simulink model "Rover_Simulation_R2023b"  (R2023b)
settings: Solver=VariableStepAuto  StartTime=0.0  StopTime=500  MaxStep=1e-1  RelTol=1e-3
values from neighbouring files (symbols this model uses):
  end_pos = [8, 7, 0]    [Mobiler_Roboter.m]
  start_pos = [1, 1, 0]    [Mobiler_Roboter.m]
undefined symbols (not defined in the file or in its folder): b, cellSize, h, l, r, r_obs, result_path, w, X_value_obs, xlim_end, Y_value_obs, ylim_end
settings Model: Creator=Asus  LastModifiedBy=sth0064
settings RTWCC: GPUComputeCapability=5.0

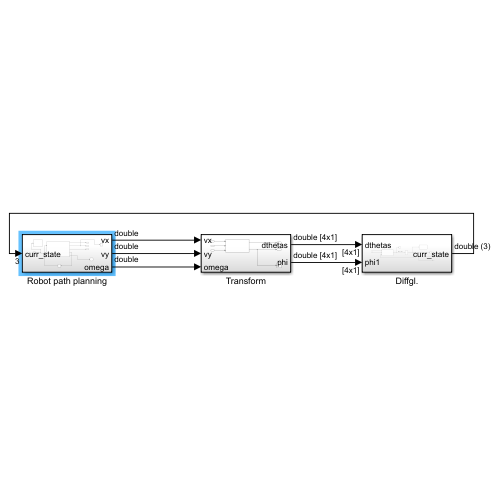
[thumbnail: Simulink's stored preview of the top-level diagram]
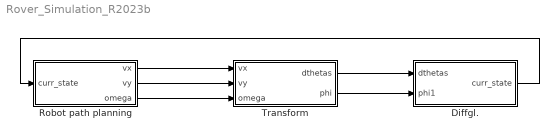
== system Rover_Simulation_R2023b ==
  Diffgl. : Subsystem
  Robot path planning : Subsystem
  Transform : Subsystem
  wires:
  Transform/1(dthetas) -> Diffgl./1(dthetas)
  Transform/2(phi) -> Diffgl./2(phi1)
  Robot path planning/1(vx) -> Transform/1(vx)
  Robot path planning/2(vy) -> Transform/2(vy)
  Diffgl./1(curr_state) -> Robot path planning/1(curr_state)
  Robot path planning/3(omega) -> Transform/3(omega)

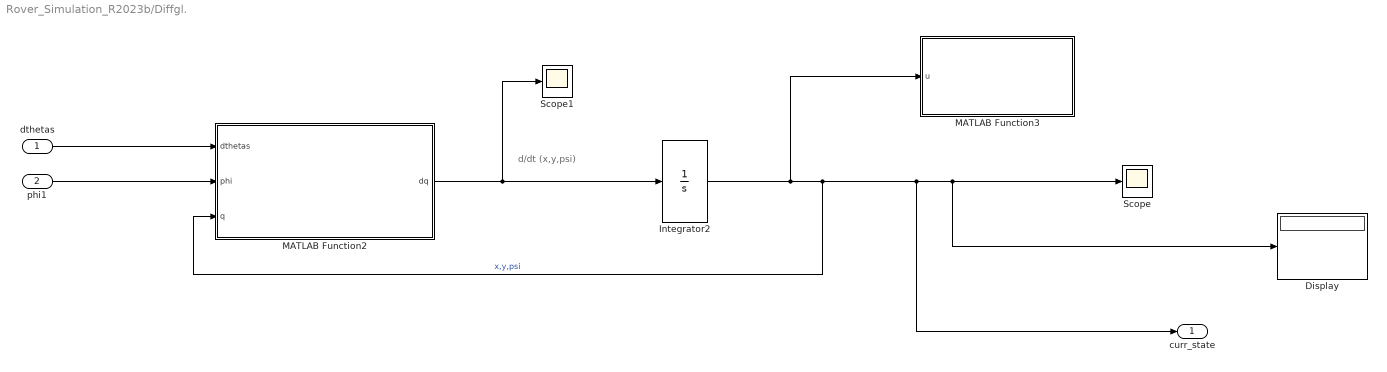
== system Rover_Simulation_R2023b/Diffgl. ==
  note: d/dt (x,y,psi)
  dthetas : Inport
  phi1 : Inport  Port=2
  Display : Display
  Integrator2 : Integrator  InitialCondition=[10;1;0]
  MATLAB Function2 : MATLAB Function  TreatAsAtomicUnit=on
  MATLAB Function3 : MATLAB Function  TreatAsAtomicUnit=on
  Scope : Scope
  Scope1 : Scope
  curr_state : Outport
  wires:
  phi1/1 -> MATLAB Function2/2(phi)
  dthetas/1 -> MATLAB Function2/1(dthetas)
  Integrator2/1 -> MATLAB Function3/1(u), curr_state/1, Display/1, Scope/1, MATLAB Function2/3(q)  "x,y,psi"
  MATLAB Function2/1(dq) -> Scope1/1, Integrator2/1

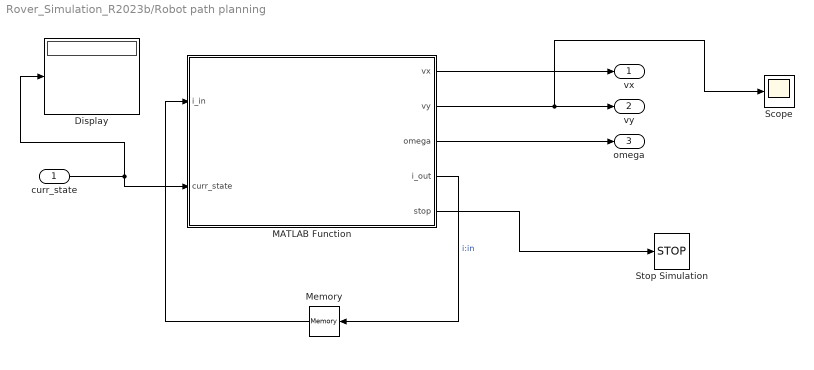
== system Rover_Simulation_R2023b/Robot path planning ==
  curr_state : Inport
  Display : Display
  MATLAB Function : MATLAB Function  TreatAsAtomicUnit=on
  Memory : Memory  InitialCondition=1  InheritSampleTime=on
  Scope : Scope
  Stop Simulation : Stop
  vx : Outport
  vy : Outport  Port=2
  omega : Outport  Port=3
  wires:
  MATLAB Function/1(vx) -> vx/1
  MATLAB Function/2(vy) -> Scope/1, vy/1
  MATLAB Function/4(i_out) -> Memory/1  "i:in"
  curr_state/1 -> Display/1, MATLAB Function/2(curr_state)
  MATLAB Function/5(stop) -> Stop Simulation/1
  Memory/1 -> MATLAB Function/1(i_in)
  MATLAB Function/3(omega) -> omega/1

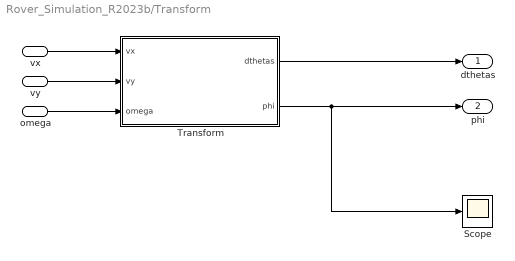
== system Rover_Simulation_R2023b/Transform ==
  vx : Inport
  vy : Inport  Port=2
  omega : Inport  Port=3
  Scope : Scope
  Transform : MATLAB Function  TreatAsAtomicUnit=on
  dthetas : Outport
  phi : Outport  Port=2
  wires:
  Transform/2(phi) -> phi/1, Scope/1
  vx/1 -> Transform/1(vx)
  Transform/1(dthetas) -> dthetas/1
  vy/1 -> Transform/2(vy)
  omega/1 -> Transform/3(omega)

== matlab function Rover_Simulation_R2023b/Transform/Transform ==
  data: vx input; vy input; omega input; dthetas output; phi output; b parameter; r parameter; l parameter
function [dthetas, phi] = fcn(vx,vy,omega, b, r, l)

vel = [vx, vy, omega];


dtheta1 = (1/r)*sqrt((vel(1) + 0.5*vel(3)*b)^2 + (vel(2)+ 0.5*vel(3)*l)^2);
dtheta2 = (1/r)*sqrt((vel(1) - 0.5*vel(3)*b)^2 + (vel(2)+ 0.5*vel(3)*l)^2);
dtheta3 = (1/r)*sqrt((vel(1) - 0.5*vel(3)*b)^2 + (vel(2) - 0.5*vel(3)*l)^2);
dtheta4 = (1/r)*sqrt((vel(1) + 0.5*vel(3)*b)^2 + (vel(2) - 0.5*vel(3)*l)^2);
    
phi1 = atan((vel(2) + vel(3) * l * 0.5) / (vel(1) + 0.5*vel(3)*b));
phi2 = atan((vel(2) + vel(3) * l * 0.5) / (vel(1) - 0.5*vel(3)*b));
phi3 = atan((vel(2) - vel(3) * l * 0.5) / (vel(1) - 0.5*vel(3)*b));
phi4 = atan((vel(2) - vel(3) * l * 0.5) / (vel(1) + 0.5*vel(3)*b));

dthetas = [dtheta1 dtheta2 dtheta3 dtheta4]';
phi = [phi1 phi2 phi3 phi4]';

end

== matlab function Rover_Simulation_R2023b/Robot path planning/MATLAB Function ==
  settings: updateMethod=DISCRETE
  data: vx output; vy output; omega output; i_out output; result_path parameter; i_in input; curr_state input; stop output; cellSize parameter
function [vx, vy, omega, i_out, stop] = P_Regler_Debug(result_path, i_in, curr_state, cellSize)
  %#codegen
  % 1) Inputs
  x   = curr_state(1);
  y   = curr_state(2);
  psi = curr_state(3);          % Heading hinzugefügt
  N   = size(result_path,1);
  stop = 0;

  
    % 2) Parameter
  Kp = 3.0 / cellSize;   % bei cellSize=0.25 → Kp_v=4.4
  Kp_omega = 3.0 / cellSize;              % Dreh-Gain
  tol = 0.4 * cellSize;    % wechselt schon bei 10 cm, wenn cellSize=0.25
  angle_tol = deg2rad(5);      % Winkel-Toleranz für reines Drehen
  v_max    = 1.0;
  
  % 3) Index clampen und Sollpunkt
  i   = max(1, min(i_in, N));
  des = result_path(i, :);     % [x_des, y_des]
  
  % 4) Fehler & Distanz
  err  = des - [x, y];
  dist = norm(err);
  psi_des = atan2(err(2), err(1));
  e_psi   = atan2(sin(psi_des - psi), cos(psi_des - psi));

  % 5) Steuerungs-Logik: Dreh-oder-Fahr
  if abs(e_psi) > angle_tol
    % zuerst drehen auf Zielrichtung
    vx    = 0;
    vy    = 0;
    omega = Kp_omega * e_psi;
  else
    % ausgerichtet: geradeaus fahren und nicht drehen
    omega = 0;
    vx = Kp * dist;
    % Begrenze Geschwindigkeit
    if vx > v_max
      vx = v_max;
    end
    vy = 0;
  end

  % 6) Waypoint-Wechsel und Stop (nur Distanz-getrieben im Body-Frame)
  % Berechne positive Vorwärtsgeschwindigkeit basierend auf Wegpunkt-Fehler
  vx = Kp * dist;
  % Begrenzung Vorwärtsgeschwindigkeit
  if vx > v_max
    vx = v_max;
  elseif vx < -v_max
    vx = -v_max;
  end
  vy = 0.01;  % lateral nicht unterstützt
  
  % 6) Omega-Regler
  psi_des = atan2(err(2), err(1));
  e_psi   = atan2(sin(psi_des - psi), cos(psi_des - psi));
  omega   = Kp_omega * e_psi;
  
  % 7) Waypoint-Wechsel und Stop
  if dist < tol && i < N
    i = i + 1;
  elseif dist < tol && i >= N
    stop = 1;
  end
  
  % 8) Outputs
  i_out    = i;
end

== matlab function Rover_Simulation_R2023b/Diffgl./MATLAB Function2 ==
  data: dthetas input; phi input; q input; r parameter; b parameter; dq output
function dq = fcn(dthetas, phi, q, r, b)

psi = q(3); 

dq = zeros(3,1);

% Rotationsmatrix
Rz = [cos(psi) -sin(psi) 0;
    sin(psi) cos(psi) 0;
    0 0 1];

% Lokale Geschwindigkeiten
vx = (r/4) * (dthetas(1)*cos(phi(1)) + dthetas(2)*cos(phi(2)) + ...
                        dthetas(3)*cos(phi(3)) + dthetas(4)*cos(phi(4))); 

vy = (r/4) * (dthetas(1)*sin(phi(1)) + dthetas(2)*sin(phi(2)) + ...
                        dthetas(3)*sin(phi(3)) + dthetas(4)*sin(phi(4)));

omega = (r/2*b) * (dthetas(1)*cos(phi(1)) - dthetas(2)*cos(phi(2)) - ...
                        dthetas(3)*cos(phi(3)) + dthetas(4)*cos(phi(4)));

roverSpeedLoc = [vx vy omega]';

dq = Rz*roverSpeedLoc;

== matlab function Rover_Simulation_R2023b/Diffgl./MATLAB Function3 ==
  settings: updateMethod=DISCRETE
  data: u input; result_path parameter; cellSize parameter; r_obs parameter; Y_value_obs parameter; X_value_obs parameter; ylim_end parameter; xlim_end parameter; end_pos parameter; start_pos parameter; l parameter; b parameter; h parameter; r parameter; w parameter
function plot_vehicle(u, result_path, cellSize, r_obs, Y_value_obs, X_value_obs, ylim_end, xlim_end, end_pos, start_pos, l, b, h, r, w)
    %#codegen
    coder.extrinsic('figure','hold','grid','axis','title', ...
                   'fct_plotvehicle','fct_plotobstacle','fct_markCircularObstacle','fct_plot_start_end', ...
                   'findobj','delete','plot','subplot','rectangle','clf','patch','quiver');

    z = 1;                  % Fahrzeughöhe
    psi = u(3);             % Yaw-Winkel

    persistent drawn;
    if isempty(drawn)
        drawn = true;
        % Initial-Setup
        figure(1); clf;
        % 3D Subplot
        subplot(1,2,1); hold on; grid on; axis equal;
        xlim([0, xlim_end]); ylim([0, ylim_end]); zlim([0,5]); title('3D-Ansicht');
        for k = 1:length(r_obs)
            fct_plotobstacle(X_value_obs(k), Y_value_obs(k), 0, r_obs(k), 1.5);
        end
        fct_plot_start_end(start_pos, end_pos);
        if ~isempty(result_path)
            for i = 1:size(result_path,1)
                plot3(result_path(i,1)*cellSize, result_path(i,2)*cellSize, z+0.1, 'b.','MarkerSize',15);
            end
        end
        % 2D Subplot
        subplot(1,2,2); hold on; grid on; axis equal;
        xlim([0, xlim_end]); ylim([0, ylim_end]); title('2D-Draufsicht');
        for k = 1:length(r_obs)
            rectangle('Position',[X_value_obs(k)-r_obs(k), Y_value_obs(k)-r_obs(k), 2*r_obs(k), 2*r_obs(k)], 'Curvature',[1,1],'EdgeColor','r');
        end
        plot(start_pos(1), start_pos(2), 'go','MarkerSize',10,'MarkerFaceColor','g');
        plot(end_pos(1), end_pos(2), 'rx','MarkerSize',10,'LineWidth',2);
        if ~isempty(result_path)
            for i = 1:size(result_path,1)
                plot(result_path(i,1)*cellSize, result_path(i,2)*cellSize, 'b.','MarkerSize',10);
            end
        end
        drawnow;
        return;
    end

    % === Update ===
    x = u(1);
    y = u(2);


    % 3D-Update (unverändert)
    subplot(1,2,1);
    old3 = findobj(gca,'Tag','vehicle'); delete(old3);
    fct_plotvehicle(x, y, z, l, b, h, r, w);

    % 2D-Update mit Orientierung
    subplot(1,2,2);
    old2 = findobj(gca,'Tag','vehicle2D'); delete(old2);
    % Rotiertes Rechteck
    corners = [l/2, b/2; -l/2, b/2; -l/2, -b/2; l/2, -b/2]';
    R = [cos(psi), -sin(psi); sin(psi), cos(psi)];
    wc = R * corners + [x; y];
    patch('XData', wc(1,:), 'YData', wc(2,:), 'FaceColor', [0.2 0.2 0.2], 'EdgeColor', 'k', 'Tag', 'vehicle2D'); hold on;
    % Heading-Pfeil
    quiver(x, y, cos(psi)*(l/2), sin(psi)*(l/2), 'MaxHeadSize',0.5, 'LineWidth',1.5, 'Color','g','Tag','vehicle2D');
    hold off;
    drawnow;
end
